simulink model "lab3_motor_model_res_load"  (R2020b)
settings: Solver=VariableStepAuto  StartTime=0.0  StopTime=10.0  RelTol=1e-3
undefined symbols (not defined in the file): Bb, Beq, daq, DiscIntNeverNeededParam, drv, gbox, Jb, Jh, mld, mot, rads2rpm, sens, tausf, Ts
libraries: simulink x1
settings Model: Creator=umberto  LastModifiedBy=Musta
settings SolverCC: AlgebraicLoopSolver=LineSearch

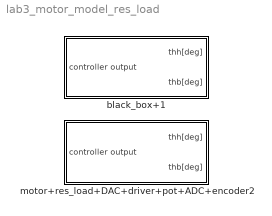
== system lab3_motor_model_res_load ==
  black_box+1 : Subsystem
  motor+res_load+DAC+driver+pot+ADC+encoder2 : Subsystem

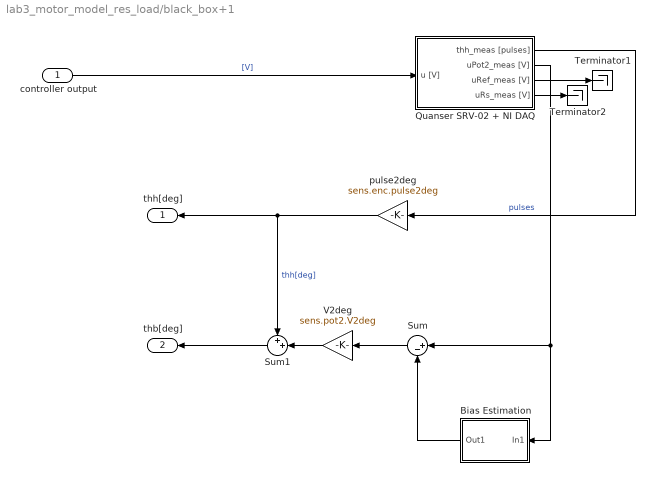
== system lab3_motor_model_res_load/black_box+1 ==
  controller output : Inport
  Bias Estimation : Subsystem
  Quanser SRV-02 + NI DAQ : Subsystem  mask(Quanser SRV-02 (with resonant load) + NI DAQ){Ts=Ts, fricType=Coulomb + viscous, lockShaft=off, beamInitPos=10}
      mask prompts: Ts "NI DAQ Sample Time:"; fricType "Friction model"; lockShaft "Lock motor shaft"; beamInitPos "Beam initial position [deg]:"
      mask help: Quanser SRV-02 (with resonant load) + NI DAQ model.
      mask init:
      | %%
      | % Riccardo Antonello (riccardo.antonello@unipd.it)
      | %
      | % April 28, 2020
      | %
      | % Dept. of Information Engineering, University of Padova
      | %
      | 
      | %%  Conversion gains
      | deg2rad = pi/180;                   %   [deg]   -> [rad]
      | rad2deg = 180/pi;                   %   [rad]   -> [deg]
      | 
      | 
      | %%  Sensors data
      | 
      | %   shunt resistor
      | sens.curr.Rs = 0.5;   
      | 
      | %   Hewlett-Packard HEDS-5540#A06 optical encoder
      | sens.enc.ppr = 500*4;                                                   %   pulses per rotation
      | sens.enc.pulse2deg = 360/sens.enc.ppr;                                  %   [pulses] -> [deg]
      | sens.enc.pulse2rad = 2*pi/sens.enc.ppr;                                 %   [pulses] -> [rad]
      | sens.enc.deg2pulse = sens.enc.ppr/360;                                  %   [deg] -> [pulses]
      | sens.enc.rad2pulse = sens.enc.ppr/2/pi;                                 %   [rad] -> [pulses]
      | 
      | %   potentiometer 2 (Spectrol 357-0-0-103) - installed on hub
      | sens.pot2.range.R      = 10e3;                                          %   ohmic value range 
      | sens.pot2.range.V      = 5;                                             %   voltage range
      | sens.pot2.range.th_deg = 340;                                           %   angle range [deg]
      | sens.pot2.range.th     = sens.pot2.range.th_deg * deg2rad;              %   angle range [rad]                           
      | sens.pot2.deg2V        = sens.pot2.range.V / sens.pot2.range.th_deg;    %   sensitivity [V/deg]
      | sens.pot2.rad2V        = sens.pot2.range.V / sens.pot2.range.th;        %   sensitivity [V/rad]
      | sens.pot2.V2deg        = 1/sens.pot2.deg2V;                             %   conversion gain [V] -> [deg]
      | sens.pot2.V2rad        = 1/sens.pot2.rad2V;                             %   conversion gain [V] -> [rad]
      | sens.pot2.noise.var    = 3.5e-7;                                        %   out noise variance [V^2]
      | 
      | 
      | %%  Data acquisition board (daq) data
      | 
      | %   NI PCI-6221 DAC data
      | daq.dac.bits = 16;                                  %   resolution (bits)
      | daq.dac.fs   = 10;                                  %   full scale 
      | daq.dac.q    = 2*daq.dac.fs/(2^daq.dac.bits-1);     %	quantization
      | 
      | %   NI PCI-6221 ADC data
      | daq.adc.bits = 16;                                  %   resolution (bits)
      | daq.adc.fs   = 10;                                  %   full scale (as set in SLDRT Analog Input block)
      | daq.adc.q    = 2*daq.adc.fs/(2^daq.adc.bits-1);     %   quantization   
      | 
      | 
      | %%  Set beam initial position
      | % SRV02Handle = find_system(gcb, ...
      | %     'LookUnderMasks', 'on', ...
      | %     'FindAll', 'on', ...
      | %     'FollowLinks', 'on', ...
      | %     'SearchDepth', '1', ...
      | %     'BlockType', 'ModelReference', ...
      | %     'Name', 'Quanser SRV-02');
      | %
      | % %get_param(SRV02Handle, 'InstanceParameters')
      | % InstanceParams = get_param(SRV02Handle, 'InstanceParameters');
      | % for k = 1:length(InstanceParams)
      | %     if strcmp(InstanceParams(k).Name, 'thb0')
      | %         if lockShaft
      | %             InstanceParams(k).Value = sprintf('%f', beamInitPos);
      | %         else
      | %             InstanceParams(k).Value = sprintf('%f', 0);    
      | %         end
      | %         set_param(SRV02Handle, 'InstanceParameters', InstanceParams);
      | %         break;
      | %     end
      | % end
      | 
      | if lockShaft
      |     thb0 = beamInitPos;
      | else
      |     thb0 = 0;    
      | end
      | 
      | 
      | %%  Mask initialization
      | if lockShaft
      |     
      |     %   find Inport handle
      |     InPortHandle = find_system(gcb, ...
      |         'LookUnderMasks', 'on', ...
      |         'FindAll', 'on', ...
      |         'FollowLinks', 'on', ...
      |         'SearchDepth', '1', ...
      |         'BlockType', 'Inport', ...
      |         'Name', 'u [V]');
      |     
      |     if ~isempty(InPortHandle)
      |     
      |         %   find DAC handle
      |         DACHandle = find_system(gcb, ...
      |             'LookUnderMasks', 'on', ...
      |             'FindAll', 'on', ...
      |             'FollowLinks', 'on', ...
      |             'SearchDepth', '1', ...
      |             'BlockType', 'SubSystem', ...
      |             'Name', 'DAC');  
      | 
      |         %   remove Inport output connection   
      |         InportConn = get_param(InPortHandle, 'PortConnectivity');
      |         delete_line(gcb, InportConn.Position);
      | 
      |         %   remove Inport block
      |         delete_block(InPortHandle);
      | 
      |         %   add Constant block
      |         ConstantHandle = add_block( ...
      |             'simulink/Sources/Constant', [gcb, '/u [V]'], ...
      |             'Position', [20   -37    50   -23], ...
      |             'Value', '0');
      | 
      |         %   connect Constant to DAC block
      |         DACPortHandles = get_param(DACHandle, 'PortHandles');
      |         ConstantPortHandles = get_param(ConstantHandle, 'PortHandles');
      |         add_line(gcb, ConstantPortHandles.Outport(1), DACPortHandles.Inport(1));
      |     
      |     end
      |     
      | else
      |     
      |     %   find Constant handle
      |     ConstantHandle = find_system(gcb, ...
      |         'LookUnderMasks', 'on', ...
      |         'FindAll', 'on', ...
      |         'FollowLinks', 'on', ...
      |         'SearchDepth', '1', ...
      |         'BlockType', 'Constant', ...
      |         'Name', 'u [V]');
      |     
      |     if ~isempty(ConstantHandle)
      |     
      |         %   find DAC handle
      |         DACHandle = find_system(gcb, ...
      |             'LookUnderMasks', 'on', ...
      |             'FindAll', 'on', ...
      |             'FollowLinks', 'on', ...
      |             'SearchDepth', '1', ...
      |             'BlockType', 'SubSystem', ...
      |             'Name', 'DAC');  
      |  
      |         %   remove Constant output connection   
      |         ConstantConn = get_param(ConstantHandle, 'PortConnectivity');
      |         delete_line(gcb, ConstantConn.Position);
      | 
      |         %   remove Inport block
      |         delete_block(ConstantHandle);   
      | 
      |         %   add Inport block
      |         InportHandle = add_block( ...
      |             'simulink/Sources/In1', [gcb, '/u [V]'], ...
      |             'Position', [20   -37    50   -23], ...
      |             'Port', '1');
      | 
      |         %   connect Constant to DAC block
      |         DACPortHandles = get_param(DACHandle, 'PortHandles');
      |         InportPortHandles = get_param(InportHandle, 'PortHandles');
      |         add_line(gcb, InportPortHandles.Outport(1), DACPortHandles.Inport(1));
      |     
      |      end
      |     
      | end
      mask Help:
      | Riccardo Antonello (antonello@dei.unipd.it)
      | 
      | April 28, 2020
      | 
      | Dept. of Information Engineering, University of Padova
      mask TypeOptions fricType: Coulomb + viscous | Karnopp
      mask Callback lockShaft:
      | %   get status of check box
      | lockShaft = get_param(gcb, 'lockShaft');
      | 
      | %   get current value of MaskVisibilities property
      | maskVisibilities = get_param(gcb, 'MaskVisibilities');
      | 
      | %   set visibility of the dialog box element
      | if strcmp(lockShaft, 'on')
      |     maskVisibilities{4} = 'on';
      | else
      |     maskVisibilities{4} = 'off';
      | end
      | 
      | % Set the 'MaskVisibilities' property for each parameter in mask
      | set_param( gcb, 'MaskVisibilities', maskVisibilities);
  Sum : Sum  Inputs=|+-
  Sum1 : Sum  Inputs=++|
  Terminator1 : Terminator
  Terminator2 : Terminator
  V2deg : Gain  Gain=sens.pot2.V2deg
  pulse2deg : Gain  Gain=sens.enc.pulse2deg
  thh[deg] : Outport
  thb[deg] : Outport  Port=2
  wires:
  Sum/1 -> V2deg/1
  Quanser SRV-02 + NI DAQ/2(uPot2_meas [V]) -> Sum/1, Bias Estimation/1(In1)
  Quanser SRV-02 + NI DAQ/4(uRs_meas [V]) -> Terminator2/1
  pulse2deg/1 -> thh[deg]/1, Sum1/1  "thh[deg]"
  Quanser SRV-02 + NI DAQ/3(uRef_meas [V]) -> Terminator1/1
  Quanser SRV-02 + NI DAQ/1(thh_meas [pulses]) -> pulse2deg/1  "pulses"
  controller output/1 -> Quanser SRV-02 + NI DAQ/1(u [V])  "[V]"
  V2deg/1 -> Sum1/2
  Sum1/1 -> thb[deg]/1
  Bias Estimation/1(Out1) -> Sum/2

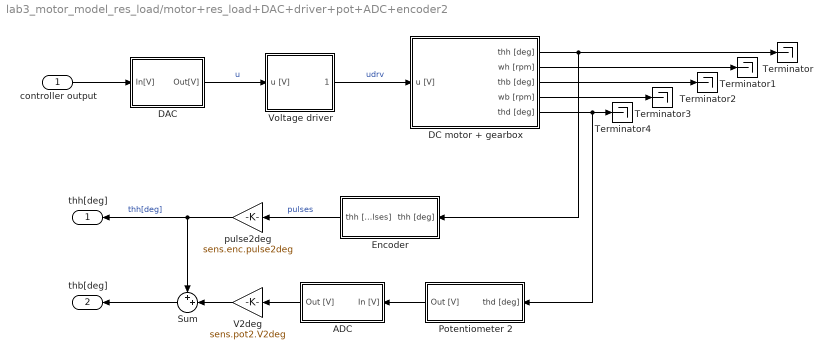
== system lab3_motor_model_res_load/motor+res_load+DAC+driver+pot+ADC+encoder2 ==
  controller output : Inport
  ADC : Subsystem
  DAC : Subsystem
  DC motor + gearbox : Subsystem
  Encoder : Subsystem
  Potentiometer 2 : Subsystem
  Sum : Sum  Inputs=++|
  Terminator{,1..4} (5 alike) : Terminator
  V2deg : Gain  Gain=sens.pot2.V2deg
  Voltage driver : Subsystem
  pulse2deg : Gain  Gain=sens.enc.pulse2deg
  thh[deg] : Outport
  thb[deg] : Outport  Port=2
  wires:
  DC motor + gearbox/4(wb [rpm]) -> Terminator3/1
  Voltage driver/1(udrv [V]) -> DC motor + gearbox/1(u [V])  "udrv"
  pulse2deg/1 -> Sum/1, thh[deg]/1  "thh[deg]"
  DC motor + gearbox/2(wh [rpm]) -> Terminator1/1
  ADC/1(Out [V]) -> V2deg/1
  V2deg/1 -> Sum/2
  DAC/1(Out[V]) -> Voltage driver/1(u [V])  "u"
  controller output/1 -> DAC/1(In[V])
  DC motor + gearbox/3(thb [deg]) -> Terminator2/1
  DC motor + gearbox/1(thh [deg]) -> Encoder/1("thh [deg] "), Terminator/1
  DC motor + gearbox/5(thd [deg]) -> Potentiometer 2/1(thd [deg]), Terminator4/1
  Potentiometer 2/1(Out [V]) -> ADC/1(In [V])
  Sum/1 -> thb[deg]/1
  Encoder/1(thh [pulses]) -> pulse2deg/1  "pulses"

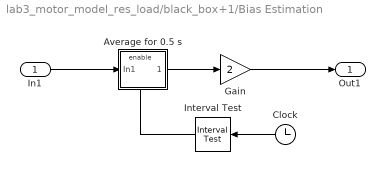
== system lab3_motor_model_res_load/black_box+1/Bias Estimation ==
  In1 : Inport
  Average for 0.5 s : Subsystem
  Clock : Clock
  Gain : Gain  Gain=2
  Interval Test : simulink/Logic and Bit Operations/Interval Test  IntervalClosedRight=on  uplimit=0.7  IntervalClosedLeft=on  lowlimit=0.2  OutDataTypeStr=boolean
  Out1 : Outport
  wires:
  Gain/1 -> Out1/1
  Average for 0.5 s/1(Out1) -> Gain/1
  Clock/1 -> Interval Test/1
  In1/1 -> Average for 0.5 s/1(In1)
  Interval Test/1 -> Average for 0.5 s/Enable

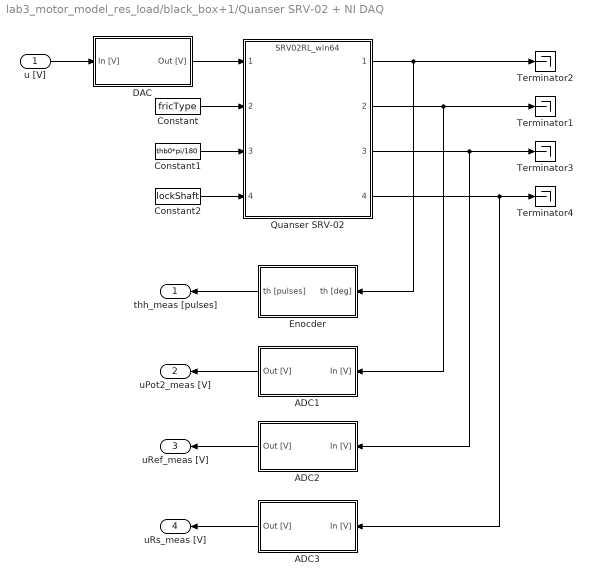
== system lab3_motor_model_res_load/black_box+1/Quanser SRV-02 + NI DAQ ==
  u [V] : Inport
  ADC1 : Subsystem
  ADC2 : Subsystem
  ADC3 : Subsystem
  Constant : Constant  Value=fricType
  Constant1 : Constant  Value=thb0*pi/180  SampleTime=Inf
  Constant2 : Constant  Value=lockShaft  SampleTime=Inf
  DAC : Subsystem
  Enocder : Subsystem
  Quanser SRV-02 : ModelReference  ModelNameDialog=SRV02RL_win64.slxp  ModelReferenceVersion=1.76  CopyOfModelProtected=on
  Terminator{1..4} (4 alike) : Terminator
  thh_meas [pulses] : Outport
  uPot2_meas [V] : Outport  Port=2
  uRef_meas [V] : Outport  Port=3
  uRs_meas [V] : Outport  Port=4
  wires:
  u [V]/1 -> DAC/1(In [V])
  ADC2/1(Out [V]) -> uRef_meas [V]/1
  Quanser SRV-02/4 -> Terminator4/1, ADC3/1(In [V])
  Constant2/1 -> Quanser SRV-02/4
  Constant1/1 -> Quanser SRV-02/3
  ADC1/1(Out [V]) -> uPot2_meas [V]/1
  Quanser SRV-02/3 -> Terminator3/1, ADC2/1(In [V])
  Constant/1 -> Quanser SRV-02/2
  Quanser SRV-02/1 -> Enocder/1(th [deg]), Terminator2/1
  Quanser SRV-02/2 -> Terminator1/1, ADC1/1(In [V])
  DAC/1(Out [V]) -> Quanser SRV-02/1
  ADC3/1(Out [V]) -> uRs_meas [V]/1
  Enocder/1(th [pulses]) -> thh_meas [pulses]/1

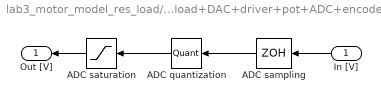
== system lab3_motor_model_res_load/motor+res_load+DAC+driver+pot+ADC+encoder2/ADC ==
  In [V] : Inport
  ADC quantization : Quantizer  QuantizationInterval=daq.adc.q
  ADC sampling : ZeroOrderHold  SampleTime=Ts
  ADC saturation : Saturate  UpperLimit=daq.adc.fs  LowerLimit=-daq.adc.fs
  Out [V] : Outport
  wires:
  ADC saturation/1 -> Out [V]/1
  ADC sampling/1 -> ADC quantization/1
  In [V]/1 -> ADC sampling/1
  ADC quantization/1 -> ADC saturation/1

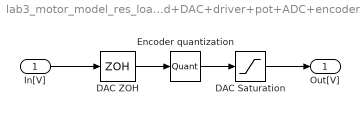
== system lab3_motor_model_res_load/motor+res_load+DAC+driver+pot+ADC+encoder2/DAC ==
  In[V] : Inport
  DAC Saturation : Saturate  UpperLimit=daq.dac.fs  LowerLimit=-daq.dac.fs  LinearizeAsGain=off
  DAC ZOH : ZeroOrderHold  SampleTime=Ts
  Encoder quantization : Quantizer  QuantizationInterval=daq.dac.q
  Out[V] : Outport
  wires:
  In[V]/1 -> DAC ZOH/1
  Encoder quantization/1 -> DAC Saturation/1
  DAC ZOH/1 -> Encoder quantization/1
  DAC Saturation/1 -> Out[V]/1

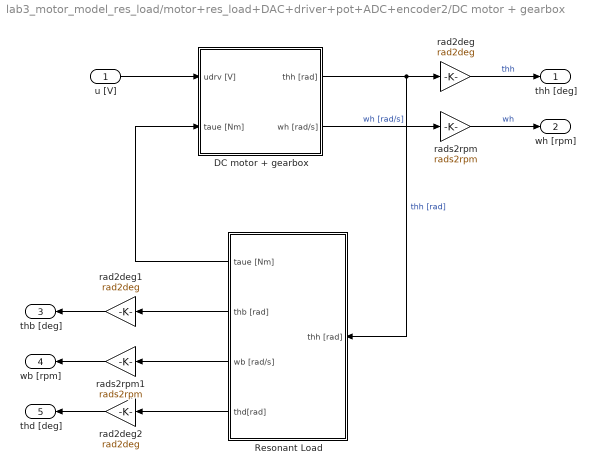
== system lab3_motor_model_res_load/motor+res_load+DAC+driver+pot+ADC+encoder2/DC motor + gearbox ==
  u [V] : Inport
  DC motor + gearbox : Subsystem
  Resonant Load : Subsystem
  rad2deg : Gain  Gain=rad2deg
  rad2deg1 : Gain  Gain=rad2deg
  rad2deg2 : Gain  Gain=rad2deg
  rads2rpm : Gain  Gain=rads2rpm
  rads2rpm1 : Gain  Gain=rads2rpm
  thh [deg] : Outport
  wh [rpm] : Outport  Port=2
  thb [deg] : Outport  Port=3
  wb [rpm] : Outport  Port=4
  thd [deg] : Outport  Port=5
  wires:
  rad2deg2/1 -> thd [deg]/1
  rads2rpm1/1 -> wb [rpm]/1
  rad2deg1/1 -> thb [deg]/1
  Resonant Load/4(thd[rad]) -> rad2deg2/1
  Resonant Load/3(wb [rad/s]) -> rads2rpm1/1
  Resonant Load/2(thb [rad]) -> rad2deg1/1
  Resonant Load/1(taue [Nm]) -> DC motor + gearbox/2(taue [Nm])
  DC motor + gearbox/1("thh [rad] ") -> Resonant Load/1(thh [rad]), rad2deg/1  "thh [rad]"
  u [V]/1 -> DC motor + gearbox/1(udrv [V])
  DC motor + gearbox/2(wh [rad/s]) -> rads2rpm/1  "wh [rad/s]"
  rad2deg/1 -> thh [deg]/1  "thh"
  rads2rpm/1 -> wh [rpm]/1  "wh"

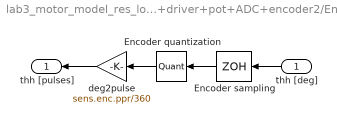
== system lab3_motor_model_res_load/motor+res_load+DAC+driver+pot+ADC+encoder2/Encoder ==
  "thh [deg] " : Inport
  Encoder quantization : Quantizer  QuantizationInterval=sens.enc.pulse2deg
  Encoder sampling : ZeroOrderHold  SampleTime=Ts
  deg2pulse : Gain  Gain=sens.enc.ppr/360
  thh [pulses] : Outport
  wires:
  "thh [deg] "/1 -> Encoder sampling/1
  Encoder sampling/1 -> Encoder quantization/1
  Encoder quantization/1 -> deg2pulse/1
  deg2pulse/1 -> thh [pulses]/1

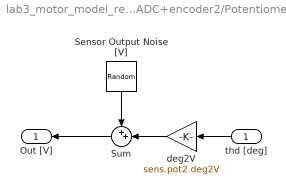
== system lab3_motor_model_res_load/motor+res_load+DAC+driver+pot+ADC+encoder2/Potentiometer 2 ==
  thd [deg] : Inport
  Sensor Output Noise [V] : RandomNumber  Variance=sens.pot2.noise.var  SampleTime=Ts
  Sum : Sum  Inputs=++|
  deg2V : Gain  Gain=sens.pot2.deg2V
  Out [V] : Outport
  wires:
  Sum/1 -> Out [V]/1
  deg2V/1 -> Sum/2
  thd [deg]/1 -> deg2V/1
  Sensor Output Noise [V]/1 -> Sum/1

== system lab3_motor_model_res_load/motor+res_load+DAC+driver+pot+ADC+encoder2/Voltage driver ==
  u [V] : Inport
  Driver dynamics : TransferFcn  Numerator=[drv.dcgain]  Denominator=[drv.Tc 1]
  Driver saturation : Saturate  UpperLimit=drv.outmax  LowerLimit=-drv.outmax  LinearizeAsGain=off
  udrv [V] : Outport
  wires:
  u [V]/1 -> Driver dynamics/1
  Driver dynamics/1 -> Driver saturation/1
  Driver saturation/1 -> udrv [V]/1

== system lab3_motor_model_res_load/black_box+1/Bias Estimation/Average for 0.5 s ==
  In1 : Inport
  Enable : EnablePort
  Discrete-Time Integrator : DiscreteIntegrator  SampleTime=Ts  ICPrevOutput=DiscIntNeverNeededParam  ICPrevScaledInput=DiscIntNeverNeededParam
  Out1 : Outport
  wires:
  Discrete-Time Integrator/1 -> Out1/1
  In1/1 -> Discrete-Time Integrator/1

== system lab3_motor_model_res_load/black_box+1/Quanser SRV-02 + NI DAQ/ADC1 ==
  In [V] : Inport
  ADC quantization : Quantizer  QuantizationInterval=daq.adc.q
  ADC sampling : ZeroOrderHold  SampleTime=Ts
  ADC saturation : Saturate  UpperLimit=daq.adc.fs  LowerLimit=-daq.adc.fs
  Out [V] : Outport
  wires:
  ADC quantization/1 -> ADC saturation/1
  In [V]/1 -> ADC sampling/1
  ADC sampling/1 -> ADC quantization/1
  ADC saturation/1 -> Out [V]/1

== system lab3_motor_model_res_load/black_box+1/Quanser SRV-02 + NI DAQ/ADC2 ==
  In [V] : Inport
  ADC quantization : Quantizer  QuantizationInterval=daq.adc.q
  ADC sampling : ZeroOrderHold  SampleTime=Ts
  ADC saturation : Saturate  UpperLimit=daq.adc.fs  LowerLimit=-daq.adc.fs
  Out [V] : Outport
  wires:
  ADC saturation/1 -> Out [V]/1
  ADC sampling/1 -> ADC quantization/1
  In [V]/1 -> ADC sampling/1
  ADC quantization/1 -> ADC saturation/1

== system lab3_motor_model_res_load/black_box+1/Quanser SRV-02 + NI DAQ/ADC3 ==
  In [V] : Inport
  Quantizer : Quantizer  QuantizationInterval=daq.adc.q
  Saturation : Saturate  UpperLimit=daq.adc.fs  LowerLimit=-daq.adc.fs
  Zero-Order Hold : ZeroOrderHold  SampleTime=Ts
  Out [V] : Outport
  wires:
  Zero-Order Hold/1 -> Quantizer/1
  Quantizer/1 -> Saturation/1
  In [V]/1 -> Zero-Order Hold/1
  Saturation/1 -> Out [V]/1

== system lab3_motor_model_res_load/black_box+1/Quanser SRV-02 + NI DAQ/DAC ==
  In [V] : Inport
  Quantizer : Quantizer  QuantizationInterval=daq.dac.q
  Saturation : Saturate  UpperLimit=daq.dac.fs  LowerLimit=-daq.dac.fs
  Zero-Order Hold : ZeroOrderHold  SampleTime=Ts
  Out [V] : Outport
  wires:
  Saturation/1 -> Out [V]/1
  Zero-Order Hold/1 -> Quantizer/1
  In [V]/1 -> Zero-Order Hold/1
  Quantizer/1 -> Saturation/1

== system lab3_motor_model_res_load/black_box+1/Quanser SRV-02 + NI DAQ/Enocder ==
  th [deg] : Inport
  Quantizer : Quantizer  QuantizationInterval=sens.enc.pulse2deg
  Zero-Order Hold : ZeroOrderHold  SampleTime=Ts
  deg2pulse : Gain  Gain=sens.enc.deg2pulse
  th [pulses] : Outport
  wires:
  deg2pulse/1 -> th [pulses]/1
  Zero-Order Hold/1 -> Quantizer/1
  th [deg]/1 -> Zero-Order Hold/1
  Quantizer/1 -> deg2pulse/1

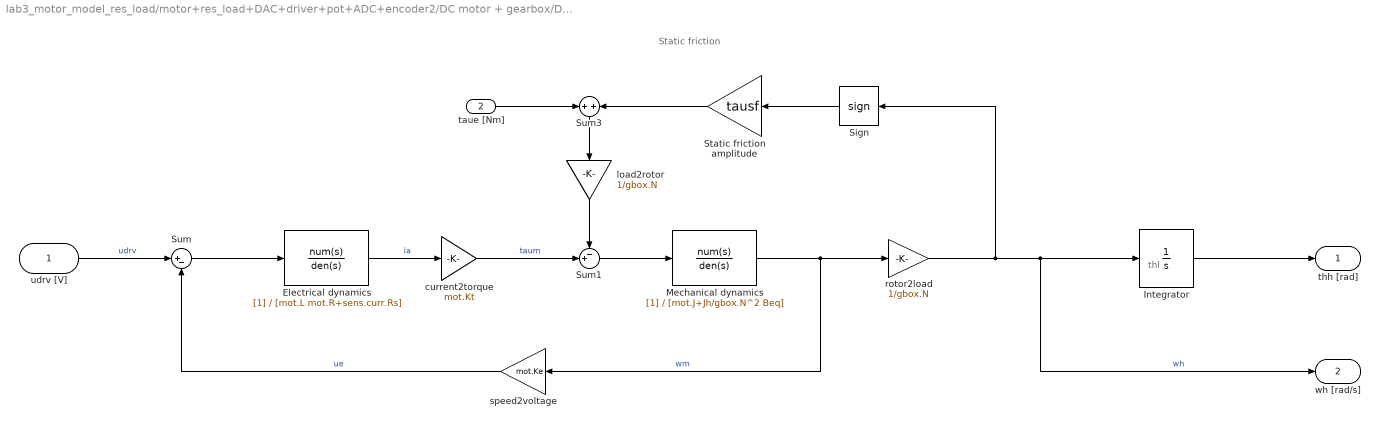
== system lab3_motor_model_res_load/motor+res_load+DAC+driver+pot+ADC+encoder2/DC motor + gearbox/DC motor + gearbox ==
  note: Static friction
  note: thl
  udrv [V] : Inport
  taue [Nm] : Inport  Port=2
  Electrical dynamics : TransferFcn  Denominator=[mot.L mot.R+sens.curr.Rs]
  Integrator : Integrator
  Mechanical dynamics : TransferFcn  Denominator=[mot.J+Jh/gbox.N^2 Beq]
  Sign : Signum  ZeroCross=off
  Static friction amplitude : Gain  Gain=tausf
  Sum : Sum  Inputs=|+-
  Sum1 : Sum  Inputs=-+|
  Sum3 : Sum  Inputs=+|+
  current2torque : Gain  Gain=mot.Kt
  load2rotor : Gain  Gain=1/gbox.N
  rotor2load : Gain  Gain=1/gbox.N
  speed2voltage : Gain  Gain=mot.Ke
  "thh [rad] " : Outport
  wh [rad/s] : Outport  Port=2
  wires:
  taue [Nm]/1 -> Sum3/1
  Static friction amplitude/1 -> Sum3/2
  Sum3/1 -> load2rotor/1
  current2torque/1 -> Sum1/2  "taum"
  load2rotor/1 -> Sum1/1
  Sum1/1 -> Mechanical dynamics/1
  Sum/1 -> Electrical dynamics/1
  rotor2load/1 -> wh [rad/s]/1, Integrator/1, Sign/1  "wh"
  Mechanical dynamics/1 -> rotor2load/1, speed2voltage/1  "wm"
  Integrator/1 -> "thh [rad] "/1
  speed2voltage/1 -> Sum/2  "ue"
  Sign/1 -> Static friction amplitude/1
  Electrical dynamics/1 -> current2torque/1  "ia"
  udrv [V]/1 -> Sum/1  "udrv"

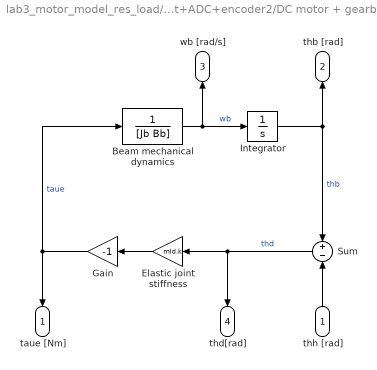
== system lab3_motor_model_res_load/motor+res_load+DAC+driver+pot+ADC+encoder2/DC motor + gearbox/Resonant Load ==
  thh [rad] : Inport
  Beam mechanical dynamics : TransferFcn  Denominator=[Jb Bb]
  Elastic joint stiffness : Gain  Gain=mld.k
  Gain : Gain  Gain=-1
  Integrator : Integrator
  Sum : Sum  Inputs=+|-
  taue [Nm] : Outport
  thb [rad] : Outport  Port=2
  wb [rad/s] : Outport  Port=3
  thd[rad] : Outport  Port=4
  wires:
  Beam mechanical dynamics/1 -> wb [rad/s]/1, Integrator/1  "wb"
  thh [rad]/1 -> Sum/2
  Integrator/1 -> thb [rad]/1, Sum/1  "thb"
  Sum/1 -> thd[rad]/1, Elastic joint stiffness/1  "thd"
  Elastic joint stiffness/1 -> Gain/1
  Gain/1 -> Beam mechanical dynamics/1, taue [Nm]/1  "taue"
